simulink model "tp_ctrlPID_sim"  (R2025b)
settings: Solver=VariableStepAuto  StartTime=0.0  StopTime=25  RelTol=1e-3
undefined symbols (not defined in the file): a, b, g, K_ol, m
libraries: simulink_extras x3
ContinueFcn:
  | tp_ctrlPID
settings Model: Creator=Francisco  LastModifiedBy=Francisco

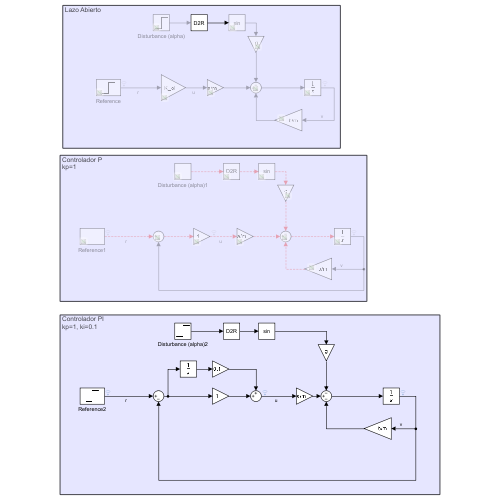
[thumbnail: Simulink's stored preview of the top-level diagram]
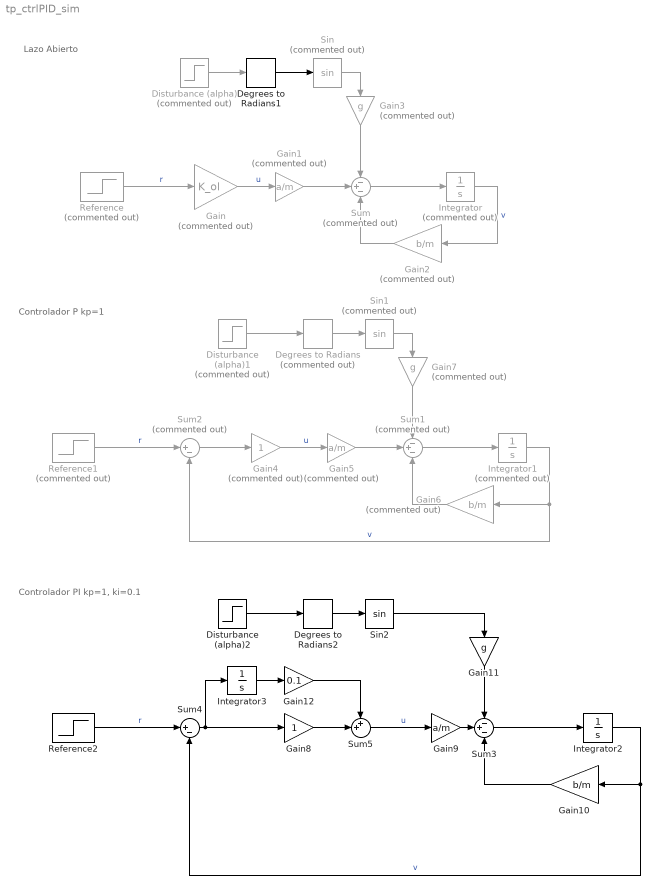
== system tp_ctrlPID_sim ==
  note: Lazo Abierto
  note: Controlador P
      | kp=1
  note: Controlador PI
      | kp=1, ki=0.1
  Degrees to Radians : simulink_extras/Transformations/Degrees to Radians  Commented=on
  Degrees to Radians1 : simulink_extras/Transformations/Degrees to Radians
  Degrees to Radians2 : simulink_extras/Transformations/Degrees to Radians
  Disturbance (alpha) : Step  Commented=on  Time=20  After=2  SampleTime=0
  Disturbance (alpha)1 : Step  Commented=on  Time=20  After=0  SampleTime=0
  Disturbance (alpha)2 : Step  Time=20  After=2  SampleTime=0
  Gain : Gain  Commented=on  Gain=K_ol
  Gain1 : Gain  Commented=on  Gain=a/m
  Gain10 : Gain  Gain=b/m
  Gain11 : Gain  Gain=g
  Gain12 : Gain  Gain=0.1
  Gain2 : Gain  Commented=on  Gain=b/m
  Gain3 : Gain  Commented=on  Gain=g
  Gain4 : Gain  Commented=on
  Gain5 : Gain  Commented=on  Gain=a/m
  Gain6 : Gain  Commented=on  Gain=b/m
  Gain7 : Gain  Commented=on  Gain=g
  Gain8 : Gain
  Gain9 : Gain  Gain=a/m
  Integrator : Integrator  Commented=on  InitialCondition=25
  Integrator1 : Integrator  Commented=on  InitialCondition=25
  Integrator2 : Integrator  InitialCondition=25
  Integrator3 : Integrator
  Reference : Step  Commented=on  Time=10  Before=25  After=35  SampleTime=0
  Reference1 : Step  Commented=on  Time=10  Before=25  After=30  SampleTime=0
  Reference2 : Step  Time=10  Before=25  After=30  SampleTime=0
  Sin : Trigonometry  Commented=on
  Sin1 : Trigonometry  Commented=on
  Sin2 : Trigonometry
  Sum : Sum  Commented=on  Inputs=-+-
  Sum1 : Sum  Commented=on  Inputs=-+-
  Sum2 : Sum  Commented=on  Inputs=|+-
  Sum3 : Sum  Inputs=-+-
  Sum4 : Sum  Inputs=|+-
  Sum5 : Sum  Inputs=++|
  wires:
  Reference/1 -> Gain/1  "r"
  Gain/1 -> Gain1/1  "u"
  Sum/1 -> Integrator/1
  Integrator/1 -> Gain2/1  "v"
  Gain2/1 -> Sum/3
  Gain1/1 -> Sum/2
  Disturbance (alpha)/1 -> Degrees to Radians1/1
  Sin/1 -> Gain3/1
  Gain3/1 -> Sum/1
  Sin1/1 -> Gain7/1
  Sum1/1 -> Integrator1/1
  Sum2/1 -> Gain4/1
  Gain7/1 -> Sum1/1
  Integrator1/1 -> Gain6/1, Sum2/2  "v"
  Gain5/1 -> Sum1/2
  Disturbance (alpha)1/1 -> Degrees to Radians/1
  Reference1/1 -> Sum2/1  "r"
  Gain6/1 -> Sum1/3
  Gain4/1 -> Gain5/1  "u"
  Degrees to Radians/1 -> Sin1/1
  Degrees to Radians1/1 -> Sin/1
  Reference2/1 -> Sum4/1  "r"
  Degrees to Radians2/1 -> Sin2/1
  Gain9/1 -> Sum3/2
  Sin2/1 -> Gain11/1
  Sum3/1 -> Integrator2/1
  Gain10/1 -> Sum3/3
  Integrator2/1 -> Gain10/1, Sum4/2  "v"
  Disturbance (alpha)2/1 -> Degrees to Radians2/1
  Gain11/1 -> Sum3/1
  Sum4/1 -> Gain8/1, Integrator3/1
  Gain8/1 -> Sum5/2
  Integrator3/1 -> Gain12/1
  Sum5/1 -> Gain9/1  "u"
  Gain12/1 -> Sum5/1
